simulink model "ms_model"  (R2019a)
settings: Solver=VariableStepAuto  StartTime=0.0  StopTime=10.0  RelTol=1e-3
undefined symbols (not defined in the file or in its folder): K, lambda
settings Model: Creator=rache  LastModifiedBy=rache

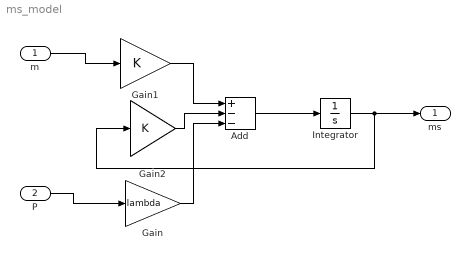
== system ms_model ==
  m : Inport
  P : Inport  Port=2
  Add : Sum  Inputs=+--
  Gain : Gain  Gain=lambda
  Gain1 : Gain  Gain=K
  Gain2 : Gain  Gain=K
  Integrator : Integrator
  ms : Outport
  wires:
  P/1 -> Gain/1
  Add/1 -> Integrator/1
  Integrator/1 -> ms/1, Gain2/1
  Gain2/1 -> Add/2
  Gain/1 -> Add/3
  Gain1/1 -> Add/1
  m/1 -> Gain1/1
